simulink model "P4p3"  (R2014a)
settings: Solver=ode1  StartTime=0.0  StopTime=25  FixedStep=0.002  RelTol=1e-3
PostLoadFcn:
  | qc_set_target_type(getConfigSet(bdroot, 'QUARC Default Target Configuration'));
values from neighbouring files (symbols this model uses):
  A = [0 1 0 0 0 0; 0 0 0 0 0 0; 0 0 0 1 0 0; 0 0 0 0 0 0; 0 0 0 0 0 1; K_3 0 0 0 0 0]    [P4p2__integral_init.m]    (also in P4p3_init.m)
  B = [0 0; 0 K_1; 0 0; K_2 0; 0 0; 0 0]    [P4p2__integral_init.m]    (also in P4p3_init.m)
  C_new = [0 0 1 0 0 0; 0 0 0 0 1 0]    [P4p3_init.m]
  Joystick_gain_x = 4    [P4p2__integral_init.m]    (also in P4p3_init.m)
  Joystick_gain_y = -7    [P4p2__integral_init.m]    (also in P4p3_init.m)
  K = lqr(A_I, B_I, Q_I, R_I)    [P4p2__integral_init.m]    (also in P4p3_init.m = lqr(A_I, B_I, Q_new, R_I))
  L_new = transpose(place(transpose(A),transpose(C_new),new_poles))    [P4p3_init.m]
  P_I = [0 9.999999999999998;9.549869109050652 0]    [P4p2__integral_init.m]    (also in P4p3_init.m)
undefined symbols (not defined in the file or in its folder): HIL, qc_get_step_size
libraries: simulink_extras x7, quarc_library x4
settings Model: SimulationMode=external  ExtModeTrigDuration=5000  Creator=Rchan  LastModifiedBy=filipga
settings SolverCC: PositivePriorityOrder=on
settings DataIOCC: SignalLoggingSaveFormat=ModelDataLogs
settings OptimizationCC: ExpressionDepthLimit=2147483647  InitFltsAndDblsToZero=on
settings DebuggingCC: SaveWithParameterizedLinksMsg=none  UnderspecifiedInitializationDetection=Classic  MultiTaskDSMMsg=warning  MultiTaskCondExecSysMsg=none  FcnCallInpInsideContextMsg=UseLocalSettings  StateNameClashWarn=warning
settings RTWCC: SystemTargetFile=quarc_win64.tlc  TemplateMakefile=quarc_default_tmf  Description=QUARC Win64 Target  ProcessScript=quarc_win64_make_rtw_hook
settings STFCustomTargetCC: CPPClassGenCompliant=on
settings GRTTargetCC: ParMdlRefBuildCompliant=off  CompOptLevelCompliant=off  CombineOutputUpdateFcns=off  MatFileLogging=off  GRTInterface=on  ExtMode=on  ExtModeMexFile=quarc_comm

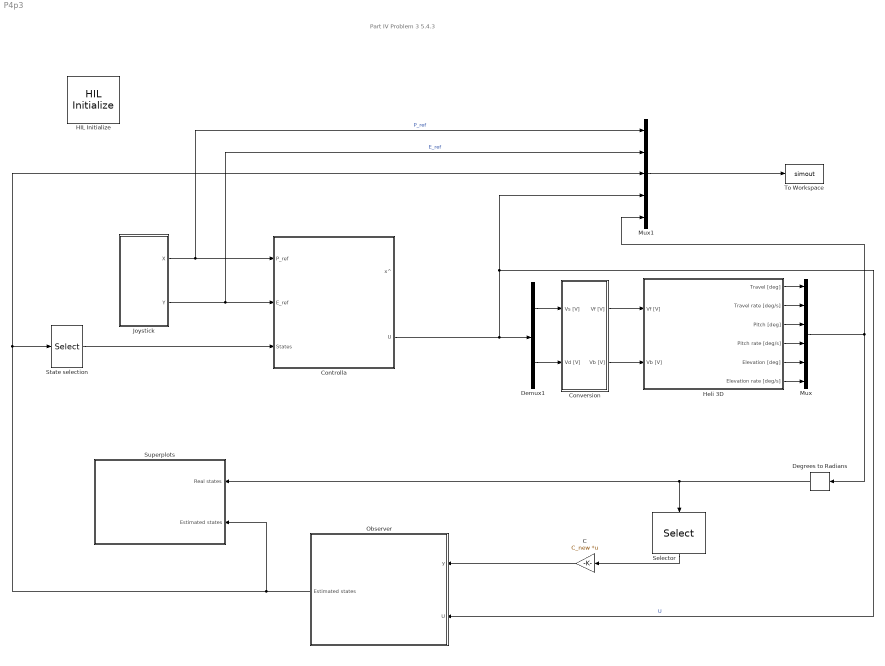
== system P4p3 ==
  note: Part IV
      | Problem 3
      | 5.4.3
  C : Gain  Gain=C_new  Multiplication=Matrix(K*u)
  Controlla : Subsystem
  Conversion : Subsystem
  Degrees to Radians : simulink_extras/Transformations/Degrees to Radians
  Demux1 : Demux  Outputs=2
  HIL Initialize : quarc_library/Data Acquisition/Generic/Configuration/HIL Initialize  Priority=-99  object_name=HIL-1  board_type=q8_usb  board_number=0  board_options=update_rate=normal;decimation=1  exclusive=off  active=off  hardware_clocks=[0:2]  clock_modes=[]  initial_clock_frequencies=[]  set_clock_params_at_start=off  set_clock_params_at_switch_in=off  set_clock_frequencies_at_start=off  set_clock_frequencies_at_switch_in=off  analog_input_channels=[0:7]  analog_input_maximums=10  analog_input_minimums=-10  set_analog_input_params_at_start=on  set_analog_input_params_at_switch_in=off  analog_output_channels=[0:7]  analog_output_maximums=10  analog_output_minimums=-10  initial_analog_outputs=[0]  final_analog_outputs=[0]  watchdog_analog_outputs=0  set_analog_output_params_at_start=on  set_analog_output_params_at_switch_in=off  set_analog_outputs_at_start=on  set_analog_outputs_at_switch_in=off  set_analog_outputs_at_terminate=on  set_analog_outputs_at_switch_out=off  set_analog_outputs_on_watchdog=off  digital_input_channels=[]  digital_output_channels=[]  digital_output_configuration=[]  initial_digital_outputs=[1]  final_digital_outputs=[1]  watchdog_digital_outputs=[1]  set_digital_output_params_at_start=off  set_digital_output_params_at_switch_in=off  set_digital_outputs_at_start=on  set_digital_outputs_at_switch_in=off  set_digital_outputs_at_terminate=on  set_digital_outputs_at_switch_out=off  set_digital_outputs_on_watchdog=off  encoder_channels=[0:7]  quadrature=[4]  encoder_filter_frequency=[]  initial_encoder_counts=[0]  set_encoder_params_at_start=on  set_encoder_params_at_switch_in=off  set_encoder_counts_at_start=on  set_encoder_counts_at_switch_in=off  pwm_channels=[0:7]  pwm_modes=0  pwm_frequency=99.532799999999995e6/4095  pwm_configuration=[0]  pwm_alignment=[0]  pwm_polarity=[1]  pwm_leading_deadband=[0]  pwm_trailing_deadband=[0]  initial_pwm_outputs=[0]  final_pwm_outputs=[0]  watchdog_pwm_outputs=[0]  set_pwm_params_at_start=on  set_pwm_params_at_switch_in=off  set_pwm_outputs_at_start=on  set_pwm_outputs_at_switch_in=off  set_pwm_outputs_at_terminate=on  set_pwm_outputs_at_switch_out=off  set_pwm_outputs_on_watchdog=off  other_output_channels=[]  initial_other_outputs=[]  final_other_outputs=[]  watchdog_other_outputs=[]  set_other_outputs_at_start=off  set_other_outputs_at_switch_in=off  set_other_outputs_at_terminate=off  set_other_outputs_at_switch_out=off  set_other_outputs_on_watchdog=off
  Heli 3D : Subsystem
  Joystick : Subsystem
  Mux : Mux  Inputs=6
  Mux1 : Mux  Inputs=5
  "Observer " : Subsystem
  Selector : Selector  InputPortWidth=6  Indices=[3 4 5 6 1 2]
  State selection : Selector  InputPortWidth=6  Indices=[1 2 4]
  Superplots : Subsystem
  To Workspace : ToWorkspace  VariableName=simout  SaveFormat=Structure With Time  SampleTime=-1
  wires:
  Conversion/2(Vb [V]) -> Heli 3D/2(Vb [V])
  Conversion/1(Vf [V]) -> Heli 3D/1(Vf [V])
  Heli 3D/1(Travel [deg]) -> Mux/1
  Heli 3D/2(Travel rate [deg/s]) -> Mux/2
  Heli 3D/3(Pitch [deg]) -> Mux/3
  Heli 3D/4(Pitch rate [deg/s]) -> Mux/4
  Heli 3D/6(Elevation rate [deg/s]) -> Mux/6
  Mux/1 -> Mux1/5, Degrees to Radians/1
  Heli 3D/5(Elevation [deg]) -> Mux/5
  Joystick/1(X) -> Mux1/1, Controlla/1(P_ref)  "P_ref"
  Joystick/2(Y) -> Mux1/2, Controlla/2(E_ref)  "E_ref"
  Degrees to Radians/1 -> Selector/1, Superplots/1(Real states)
  Controlla/2(U) -> Demux1/1, Mux1/4, "Observer "/2(U)  "U"
  Demux1/1 -> Conversion/1(Vs [V])
  Demux1/2 -> Conversion/2(Vd [V])
  Selector/1 -> C/1
  C/1 -> "Observer "/1(y)
  "Observer "/1(Estimated states) -> Superplots/2(Estimated states), Mux1/3, State selection/1
  State selection/1 -> Controlla/3(States)
  Mux1/1 -> To Workspace/1

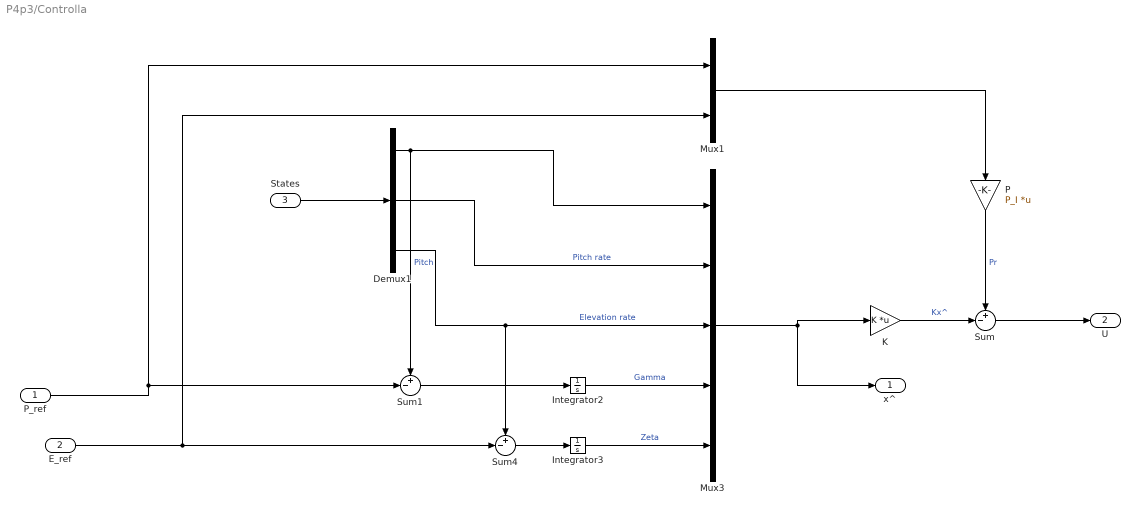
== system P4p3/Controlla ==
  P_ref : Inport
  E_ref : Inport  Port=2
  States : Inport  Port=3
  Demux1 : Demux  Outputs=3
  Integrator2 : Integrator
  Integrator3 : Integrator
  K : Gain  Gain=K  Multiplication=Matrix(K*u)
  Mux1 : Mux  Inputs=2
  Mux3 : Mux  Inputs=5
  P : Gain  Gain=P_I  Multiplication=Matrix(K*u)
  Sum : Sum  Inputs=+-|
  Sum1 : Sum  Inputs=+-|
  Sum4 : Sum  Inputs=+-|
  x^ : Outport
  U : Outport  Port=2
  wires:
  E_ref/1 -> Mux1/2, Sum4/2
  K/1 -> Sum/2  "Kx^"
  P/1 -> Sum/1  "Pr"
  Sum/1 -> U/1
  P_ref/1 -> Mux1/1, Sum1/2
  Mux1/1 -> P/1
  States/1 -> Demux1/1
  Demux1/1 -> Mux3/1, Sum1/1  "Pitch"
  Demux1/2 -> Mux3/2  "Pitch rate"
  Demux1/3 -> Sum4/1, Mux3/3  "Elevation rate"
  Sum1/1 -> Integrator2/1
  Sum4/1 -> Integrator3/1
  Integrator2/1 -> Mux3/4  "Gamma"
  Integrator3/1 -> Mux3/5  "Zeta"
  Mux3/1 -> K/1, x^/1

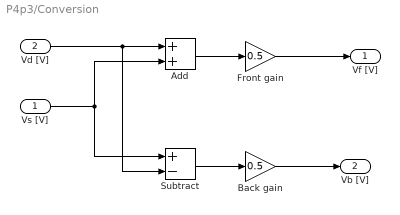
== system P4p3/Conversion ==
  Vs [V] : Inport
  Vd [V] : Inport  Port=2
  Add : Sum
  Back gain : Gain  Gain=0.5
  Front gain : Gain  Gain=0.5
  Subtract : Sum  Inputs=+-
  Vf [V] : Outport
  Vb [V] : Outport  Port=2
  wires:
  Vd [V]/1 -> Subtract/2, Add/1
  Vs [V]/1 -> Subtract/1, Add/2
  Subtract/1 -> Back gain/1
  Back gain/1 -> Vb [V]/1
  Add/1 -> Front gain/1
  Front gain/1 -> Vf [V]/1

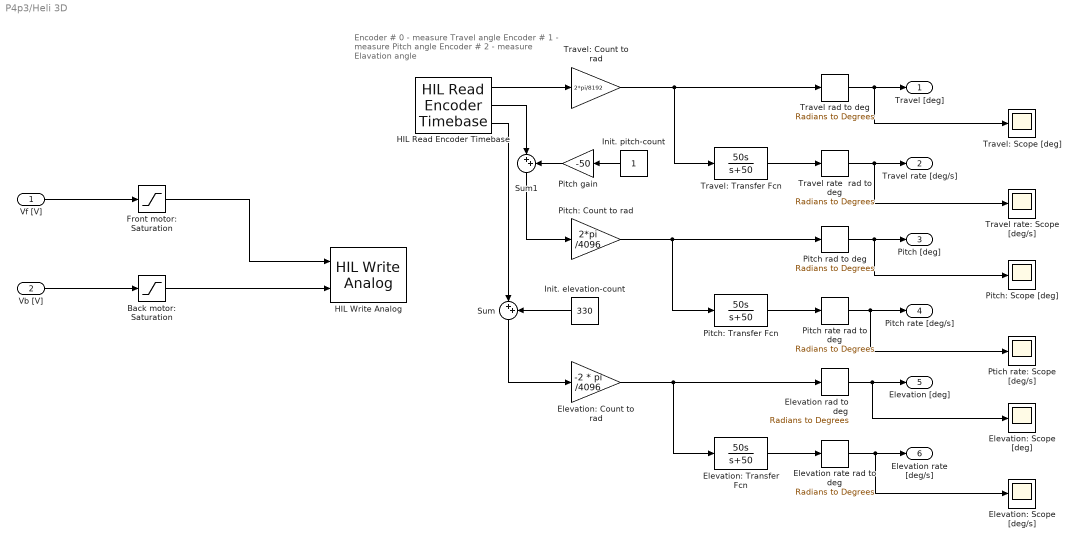
== system P4p3/Heli 3D ==
  note: Encoder # 0 - measure Travel angle
      | Encoder # 1 - measure Pitch angle
      | Encoder # 2 - measure Elavation angle
  Vf [V] : Inport
  Vb [V] : Inport  Port=2
  Back motor: Saturation : Saturate  UpperLimit=5  LowerLimit=-5
  Elevation rad to deg : simulink_extras/Transformations/Radians to Degrees
  Elevation rate rad to deg : simulink_extras/Transformations/Radians to Degrees
  Elevation: Count to rad : Gain  Gain=-2 * pi /4096
  Elevation: Scope [deg/s] : Scope
      settings: YMin=-15  YMax=15  SaveName=ScopeData13
  Elevation: Scope [deg] : Scope
      settings: YMin=-30  SaveName=ScopeData12
  Elevation: Transfer Fcn : TransferFcn  Numerator=[50 0]  Denominator=[1 50]
  Front motor: Saturation : Saturate  UpperLimit=5  LowerLimit=-5
  HIL Read Encoder Timebase : quarc_library/Data Acquisition/Generic/Timebases/HIL Read Encoder Timebase  object_name=HIL-1  clock=0  channels=[0:2]  samples_in_buffer=max(ceil(1/qc_get_step_size), 1)  active=on  vector_output=off  data_type_mode=Inherit via back propagation  data_type=double
  HIL Write Analog : quarc_library/Data Acquisition/Generic/Immediate I//O/HIL Write Analog  object_name=HIL-1  channels=[0:1]  sample_time=-1  active=off  vector_input=off
  Init. elevation-count : Constant  Value=330
  Init. pitch-count : Constant
  "Pitch gain " : Gain  Gain=-50
  Pitch rad to deg : simulink_extras/Transformations/Radians to Degrees
  Pitch rate rad to deg : simulink_extras/Transformations/Radians to Degrees
  Pitch: Count to rad : Gain  Gain=2*pi /4096
  Pitch: Scope [deg] : Scope
      settings: YMin=-60  YMax=70  SaveName=ScopeData10
  Pitch: Transfer Fcn : TransferFcn  Numerator=[50 0]  Denominator=[1 50]
  Ptich rate: Scope [deg/s] : Scope
      settings: YMin=-15  YMax=15  SaveName=ScopeData11
  Sum : Sum  Inputs=|++
  Sum1 : Sum  Inputs=|++
  Travel rad to deg : simulink_extras/Transformations/Radians to Degrees
  Travel rate  rad to deg : simulink_extras/Transformations/Radians to Degrees
  Travel rate: Scope [deg/s] : Scope
      settings: YMin=-15  YMax=15  SaveName=ScopeData9
  Travel: Count to rad : Gain  Gain=2*pi/8192
  Travel: Scope [deg] : Scope
      settings: YMin=-100  YMax=900  SaveName=ScopeData8
  Travel: Transfer Fcn : TransferFcn  Numerator=[50 0]  Denominator=[1 50]
  Travel [deg] : Outport
  Travel rate [deg/s] : Outport  Port=2
  Pitch [deg] : Outport  Port=3
  Pitch rate [deg/s] : Outport  Port=4
  Elevation [deg] : Outport  Port=5
  Elevation rate [deg/s] : Outport  Port=6
  wires:
  HIL Read Encoder Timebase/1 -> Travel: Count to rad/1
  HIL Read Encoder Timebase/2 -> Sum1/1
  Travel: Count to rad/1 -> Travel: Transfer Fcn/1, Travel rad to deg/1
  Travel: Transfer Fcn/1 -> Travel rate  rad to deg/1
  Pitch: Count to rad/1 -> Pitch: Transfer Fcn/1, Pitch rad to deg/1
  Pitch: Transfer Fcn/1 -> Pitch rate rad to deg/1
  Elevation: Count to rad/1 -> Elevation: Transfer Fcn/1, Elevation rad to deg/1
  Elevation: Transfer Fcn/1 -> Elevation rate rad to deg/1
  Travel rad to deg/1 -> Travel: Scope [deg]/1, Travel [deg]/1
  Travel rate  rad to deg/1 -> Travel rate: Scope [deg/s]/1, Travel rate [deg/s]/1
  Pitch rad to deg/1 -> Pitch [deg]/1, Pitch: Scope [deg]/1
  Pitch rate rad to deg/1 -> Ptich rate: Scope [deg/s]/1, Pitch rate [deg/s]/1
  Elevation rad to deg/1 -> Elevation: Scope [deg]/1, Elevation [deg]/1
  Elevation rate rad to deg/1 -> Elevation: Scope [deg/s]/1, Elevation rate [deg/s]/1
  Vf [V]/1 -> Front motor: Saturation/1
  Vb [V]/1 -> Back motor: Saturation/1
  Front motor: Saturation/1 -> HIL Write Analog/1
  Back motor: Saturation/1 -> HIL Write Analog/2
  HIL Read Encoder Timebase/3 -> Sum/1
  Sum/1 -> Elevation: Count to rad/1
  Init. elevation-count/1 -> Sum/2
  Init. pitch-count/1 -> "Pitch gain "/1
  Sum1/1 -> Pitch: Count to rad/1
  "Pitch gain "/1 -> Sum1/2

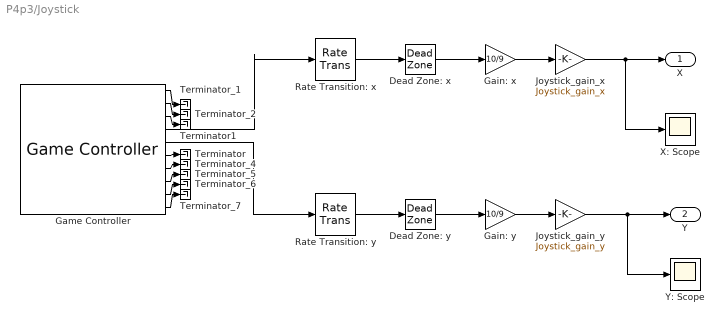
== system P4p3/Joystick ==
  Dead Zone: x : DeadZone  LowerValue=-0.1  UpperValue=0.1  SaturateOnIntegerOverflow=on
  Dead Zone: y : DeadZone  LowerValue=-0.1  UpperValue=0.1  SaturateOnIntegerOverflow=on
  Gain: x : Gain  Gain=10/9
  Gain: y : Gain  Gain=10/9
  Game Controller : quarc_library/Devices/Peripherals/Target/Game Controller  controller=1  buffer_size=12  deadzone=[]  saturation=[]  sample_time=max(qc_get_step_size, 0.01)  auto_center=off  enabled=on
  Joystick_gain_x : Gain  Gain=Joystick_gain_x
  Joystick_gain_y : Gain  Gain=Joystick_gain_y
  Rate Transition: x : RateTransition
  Rate Transition: y : RateTransition
  Terminator : Terminator
  Terminator1 : Terminator
  Terminator_{1..2,4..7} (6 alike) : Terminator
  X: Scope : Scope
      settings: YMin=-1  YMax=1  SaveName=ScopeData7
  Y: Scope : Scope
      settings: YMin=-10  YMax=10  SaveName=ScopeData5
  X : Outport
  Y : Outport  Port=2
  wires:
  Rate Transition: y/1 -> Dead Zone: y/1
  Rate Transition: x/1 -> Dead Zone: x/1
  Game Controller/5 -> Rate Transition: y/1
  Game Controller/4 -> Rate Transition: x/1
  Game Controller/1 -> Terminator_1/1
  Game Controller/2 -> Terminator_2/1
  Game Controller/7 -> Terminator_4/1
  Game Controller/8 -> Terminator_5/1
  Game Controller/9 -> Terminator_6/1
  Game Controller/10 -> Terminator_7/1
  Game Controller/3 -> Terminator1/1
  Game Controller/6 -> Terminator/1
  Dead Zone: x/1 -> Gain: x/1
  Dead Zone: y/1 -> Gain: y/1
  Gain: x/1 -> Joystick_gain_x/1
  Gain: y/1 -> Joystick_gain_y/1
  Joystick_gain_x/1 -> X/1, X: Scope/1
  Joystick_gain_y/1 -> Y: Scope/1, Y/1

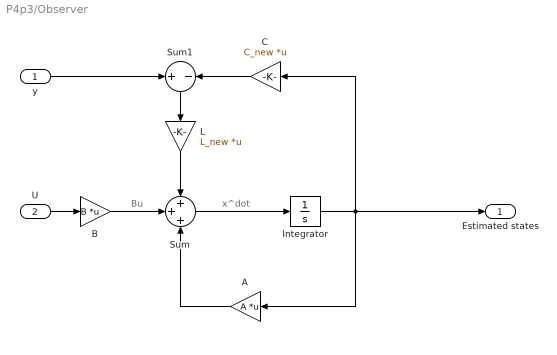
== system P4p3/Observer  ==
  note: x^dot
  note: Bu
  y : Inport
  U : Inport  Port=2
  A : Gain  Gain=A  Multiplication=Matrix(K*u)
  "B " : Gain  Gain=B  Multiplication=Matrix(K*u)
  C : Gain  Gain=C_new  Multiplication=Matrix(K*u)
  Integrator : Integrator
  L : Gain  Gain=L_new  Multiplication=Matrix(K*u)
  Sum : Sum  Inputs=+++
  Sum1 : Sum  Inputs=+|-
  Estimated states : Outport
  wires:
  Integrator/1 -> Estimated states/1, A/1, C/1
  Sum/1 -> Integrator/1
  C/1 -> Sum1/2
  L/1 -> Sum/1
  Sum1/1 -> L/1
  "B "/1 -> Sum/2
  U/1 -> "B "/1
  y/1 -> Sum1/1
  A/1 -> Sum/3

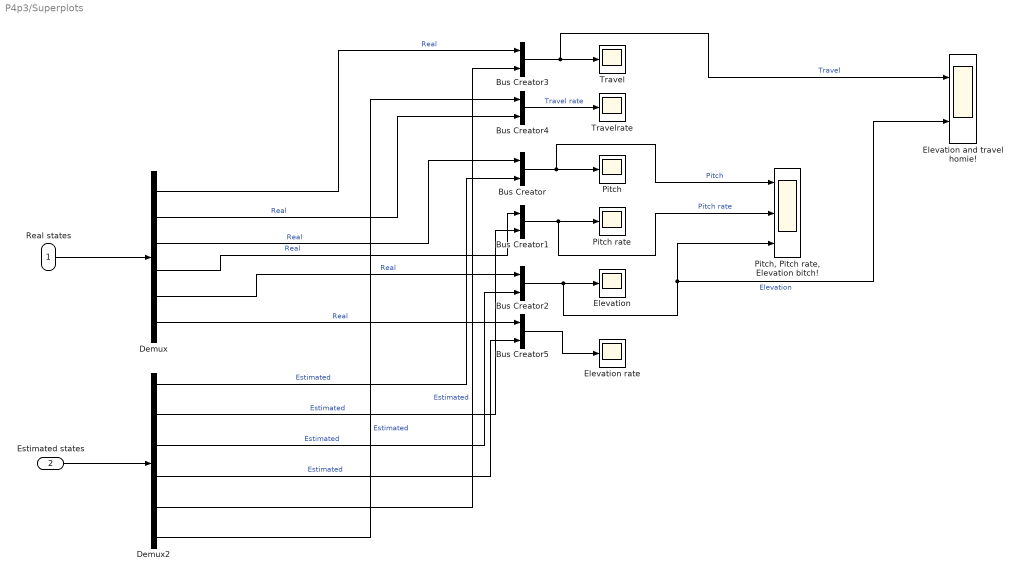
== system P4p3/Superplots ==
  Real states : Inport
  Estimated states : Inport  Port=2
  Bus Creator{,1..5} (6 alike) : BusCreator  Inputs=2
  Demux : Demux  Outputs=6
  Demux2 : Demux  Outputs=6
  Elevation : Scope
  Elevation and travel homie! : Scope  NumInputPorts=2
      settings: ShowLegends=on  YMin=-1.25~-4  YMax=1.5~2  SaveName=ScopeData3
  Elevation rate : Scope
      settings: SaveName=ScopeData6
  Pitch : Scope
  Pitch rate : Scope
      settings: SaveName=ScopeData4
  "Pitch, Pitch rate, Elevation bitch!" : Scope  NumInputPorts=3
      settings: ShowLegends=on  YMin=-1.25~-4~-0.6  YMax=1.5~2~0.45  SaveName=ScopeData15
  Travel : Scope
      settings: ShowLegends=on  SaveName=ScopeData14
  Travelrate : Scope
      settings: ShowLegends=on  SaveName=ScopeData2
  wires:
  Estimated states/1 -> Demux2/1
  Demux/3 -> Bus Creator/1  "Real"
  Bus Creator1/1 -> Pitch rate/1, "Pitch, Pitch rate, Elevation bitch!"/2  "Pitch rate"
  Demux2/5 -> Bus Creator3/2  "Estimated"
  Demux2/1 -> Bus Creator/2  "Estimated"
  Demux/6 -> Bus Creator5/1  "Real"
  Demux2/4 -> Bus Creator5/2  "Estimated"
  Real states/1 -> Demux/1
  Bus Creator/1 -> Pitch/1, "Pitch, Pitch rate, Elevation bitch!"/1  "Pitch"
  Demux2/3 -> Bus Creator2/2  "Estimated"
  Demux/1 -> Bus Creator3/1  "Real"
  Bus Creator3/1 -> Elevation and travel homie!/1, Travel/1  "Travel"
  Bus Creator5/1 -> Elevation rate/1
  Demux/5 -> Bus Creator2/1  "Real"
  Demux2/2 -> Bus Creator1/2  "Estimated"
  Demux/4 -> Bus Creator1/1  "Real"
  Bus Creator2/1 -> Elevation/1, "Pitch, Pitch rate, Elevation bitch!"/3, Elevation and travel homie!/2  "Elevation"
  Bus Creator4/1 -> Travelrate/1  "Travel rate"
  Demux2/6 -> Bus Creator4/1  "Estimated"
  Demux/2 -> Bus Creator4/2  "Real"
